simulink model "first_order_closed_loop_sim"  (R2020a)
settings: Solver=VariableStepAuto  StartTime=0.0  StopTime=30  FixedStep=1e-6  RelTol=1e-3
settings Model: Creator=Administrator  LastModifiedBy=Administrator

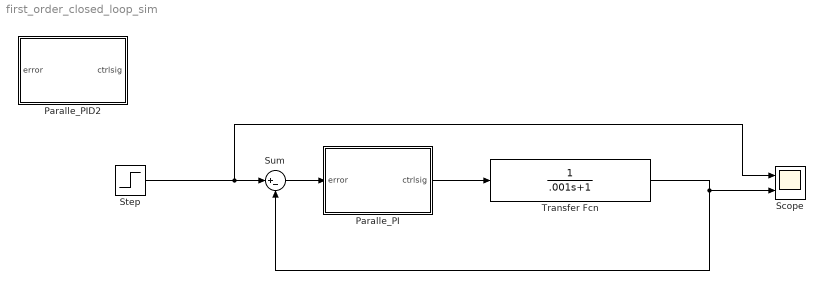
== system first_order_closed_loop_sim ==
  Paralle_PI : Subsystem
  Paralle_PID2 : Subsystem
  Scope : Scope  NumInputPorts=2
  Step : Step  SampleTime=0
  Sum : Sum  Inputs=|+-
  Transfer Fcn : TransferFcn  Denominator=[.001 1]
  wires:
  Step/1 -> Scope/1, Sum/1
  Sum/1 -> Paralle_PI/1(error)
  Transfer Fcn/1 -> Scope/2, Sum/2
  Paralle_PI/1(ctrlsig) -> Transfer Fcn/1

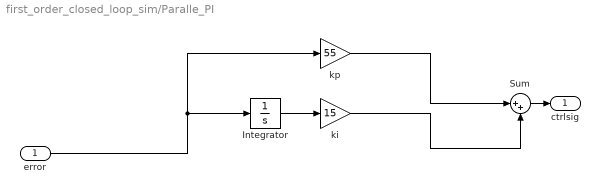
== system first_order_closed_loop_sim/Paralle_PI ==
  error : Inport
  Integrator : Integrator
  Sum : Sum  Inputs=|++
  ki : Gain  Gain=15
  kp : Gain  Gain=55
  ctrlsig : Outport
  wires:
  kp/1 -> Sum/1
  Sum/1 -> ctrlsig/1
  Integrator/1 -> ki/1
  ki/1 -> Sum/2
  error/1 -> kp/1, Integrator/1

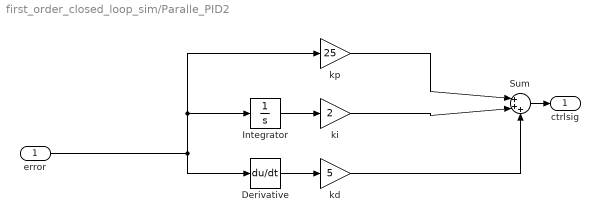
== system first_order_closed_loop_sim/Paralle_PID2 ==
  error : Inport
  Derivative : Derivative  CoefficientInTFapproximation=0
  Integrator : Integrator
  Sum : Sum  Inputs=|+++
  kd : Gain  Gain=5
  ki : Gain  Gain=2
  kp : Gain  Gain=25
  ctrlsig : Outport
  wires:
  kp/1 -> Sum/1
  kd/1 -> Sum/3
  Derivative/1 -> kd/1
  Sum/1 -> ctrlsig/1
  Integrator/1 -> ki/1
  ki/1 -> Sum/2
  error/1 -> kp/1, Integrator/1, Derivative/1
